simulink model "Plant"  (R2020b)
settings: Solver=VariableStepAuto  StartTime=0.0  StopTime=10.0  RelTol=1e-3
settings Model: Creator=hp  LastModifiedBy=hp
settings DataIOCC: SaveOutput=off  SaveTime=off

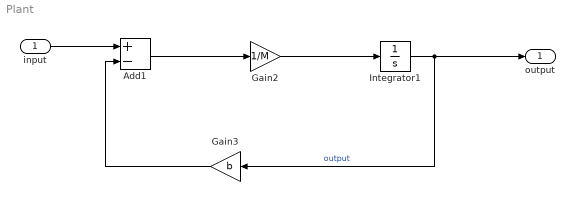
== system Plant ==
  input : Inport  OutDataTypeStr=double  PortDimensions=1
  Add1 : Sum  Inputs=+-
  Gain2 : Gain  Gain=1/M  mask{M=1000}
  Gain3 : Gain  Gain=b  mask{b=50}
  Integrator1 : Integrator
  output : Outport  OutDataTypeStr=double  PortDimensions=1  SampleTime=0
  wires:
  Gain3/1 -> Add1/2
  input/1 -> Add1/1
  Integrator1/1 -> Gain3/1, output/1  "output"
  Gain2/1 -> Integrator1/1
  Add1/1 -> Gain2/1
